simulink library "lib_energy_storage2"  (Simulink 4.1.1)
values from neighbouring files (symbols this model uses):
  logFlag = 1    [advSACompMaskInit.m]    (also in advSACompMaskInitR13.m)
undefined symbols (not defined in the file or in its folder): air_cp, amb_tmp, cyc_mph, enable_stop, ess_cap_scale, ess_cb, ess_cc, ess_coulombic_eff, ess_init_soc, ess_max_ah_cap, ess_max_p, ess_max_p_soc, ess_max_soc, ess_max_volts, ess_min_soc, ess_min_volts, ess_MMi, ess_MMo, ess_mod_airflow, ess_mod_cp, ess_mod_cpm, ess_mod_init_tmp, ess_module_mass, ess_module_num, ess_on, ess_parallel_mod_num, ess_res_scale_coef, ess_res_scale_fun, ess_set_tmp, ess_soc, ess_th_calc, ess_th_res, ess_th_res_off, ess_th_res_on, ess_tmp, ess_voc, fund_byu, fund_byuop, mc_min_volts, saber_air_temp, Saber_Battery_IO_File, saber_init_soc, saber_init_temp, saber_init_voc, saber_k_cb, saber_k_cc, saber_k_rc, saber_k_re, saber_k_rt, saber_k_soc, t_soc, time_step
libraries: simulink3 x16, lib_energy_storage x1, lib_energy_storage2 x1
(part 7 of 10)

== system lib_energy_storage2/energy storage <ess>/energy storage <ess>/Model/compute current ==
  Voc : Inport  Port=1  LatchInput=off
  Rint : Inport  Port=2  LatchInput=off
  limited output power (W) : Inport  Port=3  LatchInput=off
  Ibty=(Voc-(Voc^2-4RPbty)^.5)        ----------------------------- (2*R) : Fcn  Expr=(u[2]-(u[2]^2-4*u[1]*u[3])^.5)/(2*u[3])
  Logical Operator1 : Logic  Operator=NOT  Inputs=1
  Mux3 : Mux  Inputs=3
      settings: DisplayOption=none
  Mux4 : Mux  Inputs=3
      settings: DisplayOption=none
  Mux5 : Mux  Inputs=3
      settings: DisplayOption=none
  Voc-I*R : Fcn  Expr=u[2]-u[1]*u[3]
  enhancedToWorkspace2 : Subsystem  TreatAsAtomicUnit=on  mask(enhancedToWorkspace){generalName=generalName, specificName=current, logFlag=logFlag}
      mask prompts: generalName "General Name [char-evaluated]"; specificName "Specific Name [char-literal]"; logFlag "Enable flag (1=on,0=off)"
      mask help: A wrapper for the Simulink "To Workspace" block that allows you to evaluate the name of the variable to log to workspace. This is useful to avoid the double logging errors that occur when you pull in two library models that attempt to log to the same variable.
      mask init:
      | enhancedToWsMaker
      settings: CopyFcn=breakLinkCopyFcn  ParentCloseFcn=breakLinkParCloseFcn  RTWFcnNameOpts=Auto  RTWFileNameOpts=Auto
      mask Help:
      | <h2>Enhanced To Workspace Block</h2>
      | <h3>Parameters</h3>
      | <UL>
      | <li><b>General Name:</b> This is the more general name of the variable. Variables are saved to the workspace as <i>generalName_specificName</i>. Note that this is an evaluated variable. If you would like to type in the value directly, it must be surrounded with single quotes. Otherwise you can input the name of a variable containing a char string.</li>
      | <li><b>Specific Name:</b> This is the specific name of the variable. Note that this is input as a char literal (i.e., you don't need quotes).</li>
      | <li><b>Enable Flag:</b> This flag should have the value of 0 or 1. If 0, the variable will not be logged to the workspace. If 1, the variable will be logged. This is done so that variable logging can be turned off to improve speed.</li>
      | </ul>
      | <h3>Overview</h3>
      | <p>The enhanced to workspace block was put together to allow one to dynamically resolve variable names at run time in simulink. This is most powerful when used in conjunction with a masked subsystem to allow multiple instances of that masked subsytem to be used in the same model. The strategy is to set the generalName in the block mask which will allow the block to change the general name for all variable logging on the fly.
      | <h3>Helper Files</h3>
      | <p>Three m-files are required by the enhancedToWorkspace block. These files are located in the &lt; ADVISOR root &gt;/GUI directory :
      | <ul>
      | <li><i>enhancedToWsMaker.m</i> This file runs the mask initialization for the block</li>
      | <li><i>breakLinkCopyFcn.m</i> This file is used by the block callback when the simulink block is copied. It is necessary to break the link to the enhancedToWorkspace similar to the To Workspace block in order for it to be able to configure itself. (Try copying simulink's To Workspace block--it is impossible to make a link)</li>
      | <li><i>breakLinkParCloseFcn.m</i> This file is similar to the breakLinkCopyFcn and is used when a parent system is closed</li>
      | </ul>
      | <hr>
      | 
      | <p>Created 2003-Jan-21, Michael Patrick O'Keefe, NREL</p>
      | 
      | <!--
      | <VARDEF>
      | <H3>var_name</H3>
      | <UL>
      | <LI><B>data type</B> data type here</LI>
      | <LI><B>units</B> units here</LI>
      | <LI><B>vehicle type</B> vehicle type here</LI>
      | <LI><B>description</B> description here</LI>
      | </UL>
      | </VARDEF>
      | -->
      mask Display: disp([generalName,'_',specificName])
  ess max voltage*#batts : Constant  Value=ess_max_volts*ess_module_num
  iabs min=(Voc-Vmax)/R : Fcn  Expr=(u(1)-u(2))/u(3)
  limit current based on  max voltage during charge : Switch  Threshold=eps
  min charge current not exceeded : RelationalOperator  Operator=>
  I_ : Outport  Port=1  InitialOutput=0
  V_ : Outport  Port=2  InitialOutput=0
  tag scope: ess_maxV_limited=scoped
  wires:
  Logical Operator1/1 -> [ess_maxV_limited]
  ess max voltage*#batts/1 -> Mux5/2
  Mux5/1 -> iabs min=(Voc-Vmax)/R/1
  Mux4/1 -> Ibty=(Voc-(Voc^2-4RPbty)^.5)        ----------------------------- (2*R)/1
  Voc-I*R/1 -> V_/1
  Mux3/1 -> Voc-I*R/1
  min charge current not exceeded/1 -> Logical Operator1/1, limit current based on  max voltage during charge/2
  limit current based on  max voltage during charge/1 -> Mux3/1, I_/1, enhancedToWorkspace2/1(In1)
  iabs min=(Voc-Vmax)/R/1 -> limit current based on  max voltage during charge/3, min charge current not exceeded/2
  Ibty=(Voc-(Voc^2-4RPbty)^.5)        ----------------------------- (2*R)/1 -> limit current based on  max voltage during charge/1, min charge current not exceeded/1
  Rint/1 -> Mux5/3, Mux3/3, Mux4/3
  Voc/1 -> Mux5/1, Mux3/2, Mux4/2
  limited output power (W)/1 -> Mux4/1

== system lib_energy_storage2/energy storage <ess>/energy storage <ess>/Model/documentation9 ==

== system lib_energy_storage2/energy storage <ess>/energy storage <ess>/Model/enhancedToWorkspace ==
  In1 : Inport  Port=1  LatchInput=off
  Terminator : Terminator
  wires:
  In1/1 -> Terminator/1

== system lib_energy_storage2/energy storage <ess>/energy storage <ess>/Model/enhancedToWorkspace1 ==
  In1 : Inport  Port=1  LatchInput=off
  Terminator : Terminator
  wires:
  In1/1 -> Terminator/1

== system lib_energy_storage2/energy storage <ess>/energy storage <ess>/Model/enhancedToWorkspace2 ==
  In1 : Inport  Port=1  LatchInput=off
  Terminator : Terminator
  wires:
  In1/1 -> Terminator/1

== system lib_energy_storage2/energy storage <ess>/energy storage <ess>/Model/enhancedToWorkspace3 ==
  In1 : Inport  Port=1  LatchInput=off
  Terminator : Terminator
  wires:
  In1/1 -> Terminator/1

== system lib_energy_storage2/energy storage <ess>/energy storage <ess>/Model/enhancedToWorkspace4 ==
  In1 : Inport  Port=1  LatchInput=off
  Terminator : Terminator
  wires:
  In1/1 -> Terminator/1

== system lib_energy_storage2/energy storage <ess>/energy storage <ess>/Model/enhancedToWorkspace5 ==
  In1 : Inport  Port=1  LatchInput=off
  Terminator : Terminator
  wires:
  In1/1 -> Terminator/1

== system lib_energy_storage2/energy storage <ess>/energy storage <ess>/Model/ess tmp ==
  Qess_gen : Inport  Port=1  LatchInput=off
  Enable : EnablePort  StatesWhenEnabling=reset
  #of mods : Gain  Gain=ess_module_num  Multiplication=Element-wise(K.*u)  SaturateOnIntegerOverflow=on
  1/#of mods : Gain  Gain=1/ess_module_num  Multiplication=Element-wise(K.*u)  SaturateOnIntegerOverflow=on
  1/mcp : Gain  Gain=1/(ess_module_mass*ess_mod_cp)  Multiplication=Element-wise(K.*u)  SaturateOnIntegerOverflow=on
  Block NOTES : Subsystem
      settings: RTWFcnNameOpts=Auto  RTWFileNameOpts=Auto
      mask Display: disp('Block\nNOTES')
  Memory : Memory  Orientation=left  X0=cyc_mph(1,2)*.447  InheritSampleTime=off
      settings: RTWStateStorageClass=Auto
  Memory1 : Memory  Orientation=left  X0=cyc_mph(1,2)*.447  InheritSampleTime=off
      settings: RTWStateStorageClass=Auto
  Mux20 : Mux  Inputs=3
      settings: DisplayOption=none
  Qc : Sum  Inputs=++  SaturateOnIntegerOverflow=on
  Qess_case : Fcn  Expr=(u(2) - u(1))/u(3)
  Saturation3 : Saturate  Orientation=left  UpperLimit=1  LowerLimit=0  LinearizeAsGain=on
  Tair,ave : Subsystem  TreatAsAtomicUnit=on
      settings: RTWFcnNameOpts=Auto  RTWFileNameOpts=Auto
  Tess2 : Integrator  ExternalReset=none  InitialConditionSource=internal  InitialCondition=ess_mod_init_tmp  LimitOutput=off  UpperSaturationLimit=inf  LowerSaturationLimit=-inf  ShowSaturationPort=off  ShowStatePort=off  AbsoluteTolerance=auto
  thermostat : Fcn  Orientation=left  Expr=u(1) - ess_set_tmp
  Tess : Outport  Port=1  InitialOutput=0
  Tair : Outport  Port=2
  Qair : Outport  Port=3  OutputWhenDisabled=reset  InitialOutput=0
  wires:
  Tair,ave/1(Tair_ave) -> Tair/1, Mux20/2
  Tair,ave/2(Th Res) -> Mux20/3
  Mux20/1 -> Qess_case/1
  #of mods/1 -> Qair/1
  Memory/1 -> Tair,ave/1(Qess_case)
  Memory1/1 -> Tair,ave/Enable
  Saturation3/1 -> Memory1/1
  thermostat/1 -> Saturation3/1
  1/#of mods/1 -> Qc/2
  Qess_gen/1 -> 1/#of mods/1
  Tess2/1 -> thermostat/1, Mux20/1, Tess/1
  1/mcp/1 -> Tess2/1
  Qess_case/1 -> #of mods/1, Memory/1, Qc/1
  Qc/1 -> 1/mcp/1

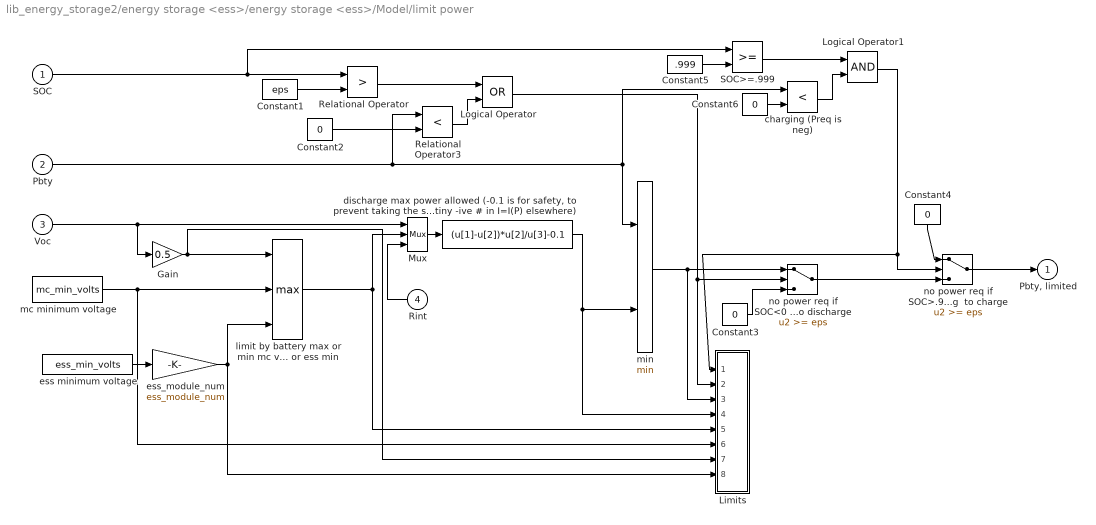
== system lib_energy_storage2/energy storage <ess>/energy storage <ess>/Model/limit power ==
  SOC : Inport  Port=1  LatchInput=off
  Pbty : Inport  Port=2  LatchInput=off
  Voc : Inport  Port=3  LatchInput=off
  Rint : Inport  Orientation=left  Port=4  LatchInput=off
  Constant1 : Constant  Value=eps
  Constant2 : Constant  Value=0
  Constant3 : Constant  Value=0
  Constant4 : Constant  Orientation=down  Value=0
  Constant5 : Constant  Value=.999
  Constant6 : Constant  Value=0
  Gain : Gain  Gain=0.5  Multiplication=Element-wise(K.*u)  SaturateOnIntegerOverflow=on
  Limits : Subsystem
      settings: RTWFcnNameOpts=Auto  RTWFileNameOpts=Auto
  Logical Operator : Logic  Operator=OR  Inputs=2
  Logical Operator1 : Logic  Operator=AND  Inputs=2
  Mux : Mux  Inputs=3
      settings: DisplayOption=none
  Relational Operator : RelationalOperator  Operator=>
  Relational Operator3 : RelationalOperator  Operator=<
  SOC>=.999 : RelationalOperator  Operator=>=
  charging (Preq is neg) : RelationalOperator  Operator=<
  "discharge max power allowed (-0.1 is for safety, to prevent taking the square of a tiny -ive # in I=I(P) elsewhere)" : Fcn  Expr=(u[1]-u[2])*u[2]/u[3]-0.1
  ess minimum voltage : Constant  Value=ess_min_volts
  ess_module_num : Gain  Gain=ess_module_num  Multiplication=Element-wise(K.*u)  SaturateOnIntegerOverflow=on
  limit by battery max or min mc voltage or ess min : MinMax  Function=max  Inputs=3
  mc minimum voltage : Constant  Value=mc_min_volts
  min : MinMax  Function=min  Inputs=2
  no power req if SOC<0 and trying  to discharge : Switch  Threshold=eps
  no power req if SOC>.999 and trying  to charge : Switch  Threshold=eps
  "Pbty, limited" : Outport  Port=1  InitialOutput=0
  wires:
  Logical Operator1/1 -> Limits/1(SOC  high limited), no power req if SOC>.999 and trying  to charge/2
  no power req if SOC>.999 and trying  to charge/1 -> "Pbty, limited"/1
  no power req if SOC<0 and trying  to discharge/1 -> no power req if SOC>.999 and trying  to charge/3
  Constant4/1 -> no power req if SOC>.999 and trying  to charge/1
  Constant5/1 -> SOC>=.999/2
  charging (Preq is neg)/1 -> Logical Operator1/2
  Constant6/1 -> charging (Preq is neg)/2
  SOC>=.999/1 -> Logical Operator1/1
  SOC/1 -> SOC>=.999/1, Relational Operator/1
  ess_module_num/1 -> Limits/8(V ess_min_volts), limit by battery max or min mc voltage or ess min/3
  ess minimum voltage/1 -> ess_module_num/1
  Gain/1 -> Limits/7(V battery (.5Voc)), limit by battery max or min mc voltage or ess min/1
  Rint/1 -> Mux/3
  mc minimum voltage/1 -> Limits/6(V mc_min_volts), limit by battery max or min mc voltage or ess min/2
  "discharge max power allowed (-0.1 is for safety, to prevent taking the square of a tiny -ive # in I=I(P) elsewhere)"/1 -> min/2, Limits/4(power bat limited)
  limit by battery max or min mc voltage or ess min/1 -> Limits/5(V used), Mux/2
  Mux/1 -> "discharge max power allowed (-0.1 is for safety, to prevent taking the square of a tiny -ive # in I=I(P) elsewhere)"/1
  min/1 -> Limits/3(power req), no power req if SOC<0 and trying  to discharge/1
  Voc/1 -> Gain/1, Mux/1
  Logical Operator/1 -> Limits/2(not SOC  low limited), no power req if SOC<0 and trying  to discharge/2
  Constant3/1 -> no power req if SOC<0 and trying  to discharge/3
  Relational Operator3/1 -> Logical Operator/2
  Constant2/1 -> Relational Operator3/2
  Pbty/1 -> charging (Preq is neg)/1, min/1, Relational Operator3/1
  Relational Operator/1 -> Logical Operator/1
  Constant1/1 -> Relational Operator/2

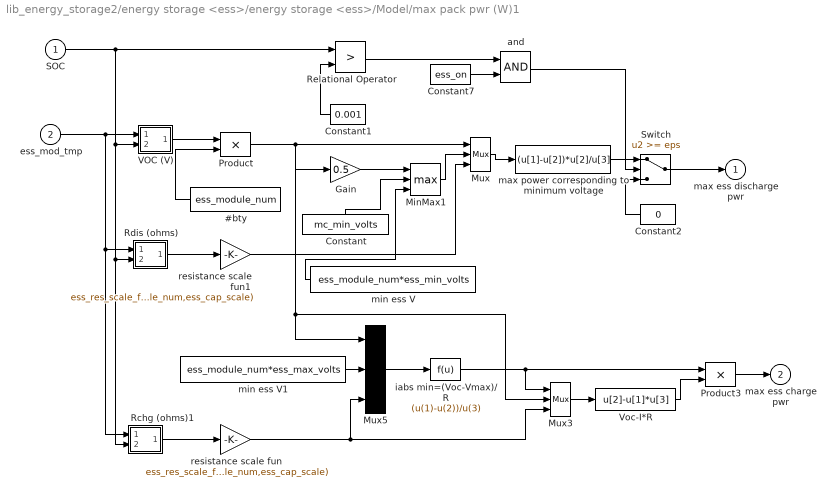
== system lib_energy_storage2/energy storage <ess>/energy storage <ess>/Model/max pack pwr (W)1 ==
  SOC : Inport  Port=1  LatchInput=off
  ess_mod_tmp : Inport  Port=2  LatchInput=off
  #bty : Constant  Orientation=left  Value=ess_module_num
  Constant : Constant  Orientation=up  Value=mc_min_volts
  Constant1 : Constant  Orientation=left  Value=0.001
  Constant2 : Constant  Orientation=left  Value=0
  Constant7 : Constant  Value=ess_on
  Gain : Gain  Gain=0.5  Multiplication=Element-wise(K.*u)  SaturateOnIntegerOverflow=on
  MinMax1 : MinMax  Function=max  Inputs=3
  Mux : Mux  Inputs=3
      settings: DisplayOption=none
  Mux3 : Mux  Inputs=3
      settings: DisplayOption=none
  Mux5 : Mux  Inputs=3
      settings: DisplayOption=none
  Product : Product  Inputs=2  Multiplication=Element-wise(.*)  SaturateOnIntegerOverflow=on
  Product3 : Product  Inputs=2  Multiplication=Element-wise(.*)  SaturateOnIntegerOverflow=on
  Rchg (ohms)1 : Subsystem  mask(2-D Table Lookup){@1=ess_tmp, @2=ess_soc, @3=ess_r_chg}
      mask prompts: @1 "X Index"; @2 "Y Index"; @3 "Table"
      mask help:
      | Two Dimensional Table Lookup
      | The first input corresponds to X Index and the second input corresponds to the Y Index
      mask init:
      | xindex=@1; yindex=@2; table=@3; sftab2chk(xindex,yindex,table);
      settings: RTWFcnNameOpts=Auto  RTWFileNameOpts=Auto
      mask Help: This block returns a linearly interpolated intersection from the table using the X index (which corresponds to the rows of the table) and the Y index (which corresponds to the columns of the table).  Extrapolation is used.
      mask Display: plot(-10,-10,110,110,[90,50,10],[90,40,30],[90,50,10],[50,26,20],[90,50,10],[22,13,10])
  Rdis (ohms) : Subsystem  mask(2-D Table Lookup){@1=ess_tmp, @2=ess_soc, @3=ess_r_dis}
      mask prompts: @1 "X Index"; @2 "Y Index"; @3 "Table"
      mask help:
      | Two Dimensional Table Lookup
      | The first input corresponds to X Index and the second input corresponds to the Y Index
      mask init:
      | xindex=@1; yindex=@2; table=@3; sftab2chk(xindex,yindex,table);
      settings: RTWFcnNameOpts=Auto  RTWFileNameOpts=Auto
      mask Help: This block returns a linearly interpolated intersection from the table using the X index (which corresponds to the rows of the table) and the Y index (which corresponds to the columns of the table).  Extrapolation is used.
      mask Display: plot(-10,-10,110,110,[90,50,10],[90,40,30],[90,50,10],[50,26,20],[90,50,10],[22,13,10])
  Relational Operator : RelationalOperator  Operator=>
  Switch : Switch  Threshold=eps
  VOC (V) : Subsystem  mask(2-D Table Lookup){@1=ess_tmp, @2=ess_soc, @3=ess_voc}
      mask prompts: @1 "X Index"; @2 "Y Index"; @3 "Table"
      mask help:
      | Two Dimensional Table Lookup
      | The first input corresponds to X Index and the second input corresponds to the Y Index
      mask init:
      | xindex=@1; yindex=@2; table=@3; sftab2chk(xindex,yindex,table);
      settings: RTWFcnNameOpts=Auto  RTWFileNameOpts=Auto
      mask Help: This block returns a linearly interpolated intersection from the table using the X index (which corresponds to the rows of the table) and the Y index (which corresponds to the columns of the table).  Extrapolation is used.
      mask Display: plot(-10,-10,110,110,[90,50,10],[90,40,30],[90,50,10],[50,26,20],[90,50,10],[22,13,10])
  Voc-I*R : Fcn  Expr=u[2]-u[1]*u[3]
  and : Logic  Operator=AND  Inputs=2
  iabs min=(Voc-Vmax)/R : Fcn  Expr=(u(1)-u(2))/u(3)
  max power corresponding to minimum voltage : Fcn  Expr=(u[1]-u[2])*u[2]/u[3]
  min ess V : Constant  Orientation=left  Value=ess_module_num*ess_min_volts
  min ess V1 : Constant  Value=ess_module_num*ess_max_volts
  resistance scale fun : Gain  Gain=ess_res_scale_fun(ess_res_scale_coef,ess_module_num,ess_cap_scale)  Multiplication=Element-wise(K.*u)  SaturateOnIntegerOverflow=on
  resistance scale fun1 : Gain  Gain=ess_res_scale_fun(ess_res_scale_coef,ess_module_num,ess_cap_scale)  Multiplication=Element-wise(K.*u)  SaturateOnIntegerOverflow=on
  max ess discharge pwr : Outport  Port=1  InitialOutput=0
  max ess charge pwr : Outport  Port=2  InitialOutput=0
  wires:
  Constant7/1 -> and/2
  Relational Operator/1 -> and/1
  and/1 -> Switch/2
  min ess V/1 -> MinMax1/3
  ess_mod_tmp/1 -> VOC (V)/1(x0), Rdis (ohms)/1(x0), Rchg (ohms)1/1(x0)
  Constant1/1 -> Relational Operator/2
  Constant/1 -> MinMax1/2
  Mux/1 -> max power corresponding to minimum voltage/1
  Gain/1 -> MinMax1/1
  MinMax1/1 -> Mux/2
  Product/1 -> Mux/1, Gain/1, Mux5/1, Mux3/2
  resistance scale fun1/1 -> Mux/3
  VOC (V)/1(table out) -> Product/1
  Rdis (ohms)/1(table out) -> resistance scale fun1/1
  max power corresponding to minimum voltage/1 -> Switch/1
  Constant2/1 -> Switch/3
  SOC/1 -> Relational Operator/1, VOC (V)/2(y0), Rdis (ohms)/2(y0), Rchg (ohms)1/2(y0)
  Switch/1 -> max ess discharge pwr/1
  min ess V1/1 -> Mux5/2
  Mux5/1 -> iabs min=(Voc-Vmax)/R/1
  Mux3/1 -> Voc-I*R/1
  iabs min=(Voc-Vmax)/R/1 -> Mux3/1, Product3/1
  Voc-I*R/1 -> Product3/2
  Product3/1 -> max ess charge pwr/1
  resistance scale fun/1 -> Mux5/3, Mux3/3
  Rchg (ohms)1/1(table out) -> resistance scale fun/1
  #bty/1 -> Product/2

== system lib_energy_storage2/energy storage <ess>/energy storage <ess>/Model/pack Voc, Rint ==
  SOC (prev) : Inport  Port=1  LatchInput=off
  req'd battery power (W) : Inport  Port=2  LatchInput=off
  mod tmp   (C) : Inport  Port=3  LatchInput=off
  #bty : Constant  Value=ess_module_num
  Product : Product  Inputs=2  Multiplication=Element-wise(.*)  SaturateOnIntegerOverflow=on
  Rchg (ohms) : Subsystem  mask(2-D Table Lookup){@1=ess_tmp, @2=ess_soc, @3=ess_r_chg}
      mask prompts: @1 "X Index"; @2 "Y Index"; @3 "Table"
      mask help:
      | Two Dimensional Table Lookup
      | The first input corresponds to X Index and the second input corresponds to the Y Index
      mask init:
      | xindex=@1; yindex=@2; table=@3; sftab2chk(xindex,yindex,table);
      settings: RTWFcnNameOpts=Auto  RTWFileNameOpts=Auto
      mask Help: This block returns a linearly interpolated intersection from the table using the X index (which corresponds to the rows of the table) and the Y index (which corresponds to the columns of the table).  Extrapolation is used.
      mask Display: plot(-10,-10,110,110,[90,50,10],[90,40,30],[90,50,10],[50,26,20],[90,50,10],[22,13,10])
  Rdis (ohms) : Subsystem  mask(2-D Table Lookup){@1=ess_tmp, @2=ess_soc, @3=ess_r_dis}
      mask prompts: @1 "X Index"; @2 "Y Index"; @3 "Table"
      mask help:
      | Two Dimensional Table Lookup
      | The first input corresponds to X Index and the second input corresponds to the Y Index
      mask init:
      | xindex=@1; yindex=@2; table=@3; sftab2chk(xindex,yindex,table);
      settings: RTWFcnNameOpts=Auto  RTWFileNameOpts=Auto
      mask Help: This block returns a linearly interpolated intersection from the table using the X index (which corresponds to the rows of the table) and the Y index (which corresponds to the columns of the table).  Extrapolation is used.
      mask Display: plot(-10,-10,110,110,[90,50,10],[90,40,30],[90,50,10],[50,26,20],[90,50,10],[22,13,10])
  Switch : Switch  Threshold=0
  VOC (V) : Subsystem  mask(2-D Table Lookup){@1=ess_tmp, @2=ess_soc, @3=ess_voc}
      mask prompts: @1 "X Index"; @2 "Y Index"; @3 "Table"
      mask help:
      | Two Dimensional Table Lookup
      | The first input corresponds to X Index and the second input corresponds to the Y Index
      mask init:
      | xindex=@1; yindex=@2; table=@3; sftab2chk(xindex,yindex,table);
      settings: RTWFcnNameOpts=Auto  RTWFileNameOpts=Auto
      mask Help: This block returns a linearly interpolated intersection from the table using the X index (which corresponds to the rows of the table) and the Y index (which corresponds to the columns of the table).  Extrapolation is used.
      mask Display: plot(-10,-10,110,110,[90,50,10],[90,40,30],[90,50,10],[50,26,20],[90,50,10],[22,13,10])
  resistance scale fun : Gain  Gain=ess_res_scale_fun(ess_res_scale_coef,ess_module_num,ess_cap_scale)  Multiplication=Element-wise(K.*u)  SaturateOnIntegerOverflow=on
  resistance scale fun1 : Gain  Gain=ess_res_scale_fun(ess_res_scale_coef,ess_module_num,ess_cap_scale)  Multiplication=Element-wise(K.*u)  SaturateOnIntegerOverflow=on
  pack open- circuit voltage : Outport  Port=1  InitialOutput=0
  pack resistance : Outport  Port=2  InitialOutput=0
  wires:
  mod tmp   (C)/1 -> Rchg (ohms)/1(x0), Rdis (ohms)/1(x0), VOC (V)/1(x0)
  SOC (prev)/1 -> Rchg (ohms)/2(y0), Rdis (ohms)/2(y0), VOC (V)/2(y0)
  req'd battery power (W)/1 -> Switch/2
  VOC (V)/1(table out) -> Product/1
  Product/1 -> pack open- circuit voltage/1
  #bty/1 -> Product/2
  Switch/1 -> pack resistance/1
  Rdis (ohms)/1(table out) -> resistance scale fun/1
  resistance scale fun/1 -> Switch/1
  Rchg (ohms)/1(table out) -> resistance scale fun1/1
  resistance scale fun1/1 -> Switch/3

== system lib_energy_storage2/energy storage <ess>/energy storage <ess>/Model/stop sim ==
  SOC : Inport  Port=1  LatchInput=off
  Enable : EnablePort
  Const : Constant  Orientation=up  Value=.001
  Relational Operator : RelationalOperator  Operator=<
  Stop Simulation : Stop
  wires:
  Relational Operator/1 -> Stop Simulation/1
  SOC/1 -> Relational Operator/1
  Const/1 -> Relational Operator/2

== system lib_energy_storage2/energy storage <ess> RC/energy storage <ess> RC/model/Allow simulation to stop based on  low SOC ==
  SOC : Inport  Port=1  LatchInput=off
  Enable : EnablePort
  Const : Constant  Orientation=up  Value=.001
  Relational Operator : RelationalOperator  Operator=<
  Stop Simulation : Stop
  wires:
  Relational Operator/1 -> Stop Simulation/1
  SOC/1 -> Relational Operator/1
  Const/1 -> Relational Operator/2

== system lib_energy_storage2/energy storage <ess> RC/energy storage <ess> RC/model/Block NOTES ==
  note: This block models the energy storage system as an SOC-dependent voltage
      | in series with an SOC- and current direction-dependent internal resistance.
      | SOC is computed assuming that A-h capacity is constant, but limited
      | such that a minimum voltage is never exceeded (replacing the
      | previous Peukert relationship which underpredicted battery capacity).
      |
      | Discharge power is limited here so as not to bring the bus (battery pack) voltage below
      | the minimum controller voltage or the minimum battery voltage and so as to allow
      | the solution of the quadratic eq'n for discharge current.
      |
      | Charge current is limited to ensure the voltage does not exceed a maximum
      | voltage
      |
      | Positive current is discharge current in the convention used here.
      | Power loss is computed as I*R+losses due to Coulombic (in)efficiency.
      |
      | Thermal modeling of the battery performance is modeled in the
      | OCV, Rint, and capacity.

== system lib_energy_storage2/energy storage <ess> RC/energy storage <ess> RC/model/Model Parameters ==
  SOC : Inport  Port=1  LatchInput=off
  Ess Temp : Inport  Port=2  LatchInput=off
  Preq : Inport  Port=3  LatchInput=off
  Terminator : Terminator
  cb : Lookup  InputValues=ess_tmp  OutputValues=ess_cb
  cc : Lookup  InputValues=ess_tmp  OutputValues=ess_cc
  rc : Subsystem  mask(2-D Table Lookup){@1=ess_tmp, @2=ess_soc, @3=ess_rc}
      mask prompts: @1 "X Index"; @2 "Y Index"; @3 "Table"
      mask help:
      | Two Dimensional Table Lookup
      | The first input corresponds to X Index and the second input corresponds to the Y Index
      mask init:
      | xindex=@1; yindex=@2; table=@3; sftab2chk(xindex,yindex,table);
      settings: RTWFcnNameOpts=Auto  RTWFileNameOpts=Auto
      mask Help: This block returns a linearly interpolated intersection from the table using the X index (which corresponds to the rows of the table) and the Y index (which corresponds to the columns of the table).  Extrapolation is used.
      mask Display: plot(-10,-10,110,110,[90,50,10],[90,40,30],[90,50,10],[50,26,20],[90,50,10],[22,13,10])
  re : Subsystem  mask(2-D Table Lookup){@1=ess_tmp, @2=ess_soc, @3=ess_re}
      mask prompts: @1 "X Index"; @2 "Y Index"; @3 "Table"
      mask help:
      | Two Dimensional Table Lookup
      | The first input corresponds to X Index and the second input corresponds to the Y Index
      mask init:
      | xindex=@1; yindex=@2; table=@3; sftab2chk(xindex,yindex,table);
      settings: RTWFcnNameOpts=Auto  RTWFileNameOpts=Auto
      mask Help: This block returns a linearly interpolated intersection from the table using the X index (which corresponds to the rows of the table) and the Y index (which corresponds to the columns of the table).  Extrapolation is used.
      mask Display: plot(-10,-10,110,110,[90,50,10],[90,40,30],[90,50,10],[50,26,20],[90,50,10],[22,13,10])
  rt : Subsystem  mask(2-D Table Lookup){@1=ess_tmp, @2=ess_soc, @3=ess_rt}
      mask prompts: @1 "X Index"; @2 "Y Index"; @3 "Table"
      mask help:
      | Two Dimensional Table Lookup
      | The first input corresponds to X Index and the second input corresponds to the Y Index
      mask init:
      | xindex=@1; yindex=@2; table=@3; sftab2chk(xindex,yindex,table);
      settings: RTWFcnNameOpts=Auto  RTWFileNameOpts=Auto
      mask Help: This block returns a linearly interpolated intersection from the table using the X index (which corresponds to the rows of the table) and the Y index (which corresponds to the columns of the table).  Extrapolation is used.
      mask Display: plot(-10,-10,110,110,[90,50,10],[90,40,30],[90,50,10],[50,26,20],[90,50,10],[22,13,10])
  Cb : Outport  Port=1  InitialOutput=0
  Cc : Outport  Port=2  InitialOutput=0
  Re : Outport  Port=3  InitialOutput=0
  Rc : Outport  Port=4  InitialOutput=0
  Rt : Outport  Port=5  InitialOutput=0
  wires:
  rc/1(table out) -> Rc/1
  rt/1(table out) -> Rt/1
  re/1(table out) -> Re/1
  cc/1 -> Cc/1
  cb/1 -> Cb/1
  SOC/1 -> rt/2(y0), rc/2(y0), re/2(y0)
  Preq/1 -> Terminator/1
  Ess Temp/1 -> rt/1(x0), rc/1(x0), re/1(x0), cc/1, cb/1

== system lib_energy_storage2/energy storage <ess> RC/energy storage <ess> RC/model/RC model ==
  Cb : Inport  Port=1  LatchInput=off
  Cc : Inport  Port=2  LatchInput=off
  Re : Inport  Port=3  LatchInput=off
  Rc : Inport  Port=4  LatchInput=off
  Rt : Inport  Port=5  LatchInput=off
  Preq : Inport  Port=6  LatchInput=off
  Ess Temp : Inport  Port=7  LatchInput=off
  #mods{,1..4} (5 alike) : Gain  Gain=ess_module_num  Multiplication=Element-wise(K.*u)  SaturateOnIntegerOverflow=on
  1/#mods : Gain  Gain=1/ess_module_num  Multiplication=Element-wise(K.*u)  SaturateOnIntegerOverflow=on
  Demux1 : Demux  Outputs=7  BusSelectionMode=off
  Memory1 : Memory  X0=ess_init_soc  InheritSampleTime=off
      settings: RTWStateStorageClass=Auto
  Memory2 : Memory  X0=0  InheritSampleTime=off
      settings: RTWStateStorageClass=Auto
  Memory3 : Memory  X0=0  InheritSampleTime=off
      settings: RTWStateStorageClass=Auto
  Mux2 : Mux  Inputs=7
      settings: DisplayOption=none
  RC model of one module : S-Function  FunctionName=RC  Parameters=ess_min_volts,ess_max_volts,mc_min_volts/ess_module_num,ess_soc,ess_tmp,ess_voc,ess_init_soc,ess_mod_init_tmp  PortCounts=[]  SFunctionModules=''
  enhancedToWorkspace6 : Subsystem  TreatAsAtomicUnit=on  mask(enhancedToWorkspace){generalName=generalName, specificName=current, logFlag=logFlag}
      mask prompts: generalName "General Name [char-evaluated]"; specificName "Specific Name [char-literal]"; logFlag "Enable flag (1=on,0=off)"
      mask help: A wrapper for the Simulink "To Workspace" block that allows you to evaluate the name of the variable to log to workspace. This is useful to avoid the double logging errors that occur when you pull in two library models that attempt to log to the same variable.
      mask init:
      | enhancedToWsMaker
      settings: CopyFcn=breakLinkCopyFcn  ParentCloseFcn=breakLinkParCloseFcn  RTWFcnNameOpts=Auto  RTWFileNameOpts=Auto
      mask Help:
      | <h2>Enhanced To Workspace Block</h2>
      | <h3>Parameters</h3>
      | <UL>
      | <li><b>General Name:</b> This is the more general name of the variable. Variables are saved to the workspace as <i>generalName_specificName</i>. Note that this is an evaluated variable. If you would like to type in the value directly, it must be surrounded with single quotes. Otherwise you can input the name of a variable containing a char string.</li>
      | <li><b>Specific Name:</b> This is the specific name of the variable. Note that this is input as a char literal (i.e., you don't need quotes).</li>
      | <li><b>Enable Flag:</b> This flag should have the value of 0 or 1. If 0, the variable will not be logged to the workspace. If 1, the variable will be logged. This is done so that variable logging can be turned off to improve speed.</li>
      | </ul>
      | <h3>Overview</h3>
      | <p>The enhanced to workspace block was put together to allow one to dynamically resolve variable names at run time in simulink. This is most powerful when used in conjunction with a masked subsystem to allow multiple instances of that masked subsytem to be used in the same model. The strategy is to set the generalName in the block mask which will allow the block to change the general name for all variable logging on the fly.
      | <h3>Helper Files</h3>
      | <p>Three m-files are required by the enhancedToWorkspace block. These files are located in the &lt; ADVISOR root &gt;/GUI directory :
      | <ul>
      | <li><i>enhancedToWsMaker.m</i> This file runs the mask initialization for the block</li>
      | <li><i>breakLinkCopyFcn.m</i> This file is used by the block callback when the simulink block is copied. It is necessary to break the link to the enhancedToWorkspace similar to the To Workspace block in order for it to be able to configure itself. (Try copying simulink's To Workspace block--it is impossible to make a link)</li>
      | <li><i>breakLinkParCloseFcn.m</i> This file is similar to the breakLinkCopyFcn and is used when a parent system is closed</li>
      | </ul>
      | <hr>
      | 
      | <p>Created 2003-Jan-21, Michael Patrick O'Keefe, NREL</p>
      | 
      | <!--
      | <VARDEF>
      | <H3>var_name</H3>
      | <UL>
      | <LI><B>data type</B> data type here</LI>
      | <LI><B>units</B> units here</LI>
      | <LI><B>vehicle type</B> vehicle type here</LI>
      | <LI><B>description</B> description here</LI>
      | </UL>
      | </VARDEF>
      | -->
      mask Display: disp([generalName,'_',specificName])
  Pavailable : Outport  Port=1  InitialOutput=0
  SOC : Outport  Port=2  InitialOutput=0
  Vout : Outport  Port=3  InitialOutput=0
  Qess_gen : Outport  Port=4  InitialOutput=0
  tag scope: ess_max_chg_pwr=scoped, ess_max_pwr=scoped
  wires:
  RC model of one module/1 -> Demux1/1
  #mods2/1 -> Qess_gen/1
  Demux1/4 -> #mods2/1
  #mods1/1 -> Vout/1
  Demux1/3 -> #mods1/1
  #mods/1 -> Pavailable/1
  Demux1/1 -> #mods/1
  1/#mods/1 -> Mux2/6
  Preq/1 -> 1/#mods/1
  Mux2/1 -> RC model of one module/1
  Rt/1 -> Mux2/5
  Rc/1 -> Mux2/4
  Re/1 -> Mux2/3
  Cc/1 -> Mux2/2
  Cb/1 -> Mux2/1
  Ess Temp/1 -> Mux2/7
  Demux1/7 -> enhancedToWorkspace6/1(In1)
  Demux1/6 -> #mods4/1
  Memory2/1 -> [ess_max_chg_pwr]
  Demux1/5 -> #mods3/1
  Memory3/1 -> [ess_max_pwr]
  Demux1/2 -> Memory1/1
  Memory1/1 -> SOC/1
  #mods3/1 -> Memory3/1
  #mods4/1 -> Memory2/1

== system lib_energy_storage2/energy storage <ess> RC/energy storage <ess> RC/model/Thermal Model of Battery ==
  Qess_gen : Inport  Port=1  LatchInput=off
  Enable : EnablePort  StatesWhenEnabling=reset
  #of mods : Gain  Gain=ess_module_num  Multiplication=Element-wise(K.*u)  SaturateOnIntegerOverflow=on
  1/#of mods : Gain  Gain=1/ess_module_num  Multiplication=Element-wise(K.*u)  SaturateOnIntegerOverflow=on
  1/mcp : Gain  Gain=1/(ess_module_mass*ess_mod_cp)  Multiplication=Element-wise(K.*u)  SaturateOnIntegerOverflow=on
  Block NOTES : Subsystem
      settings: RTWFcnNameOpts=Auto  RTWFileNameOpts=Auto
      mask Display: disp('Block\nNOTES')
  Memory : Memory  Orientation=left  X0=cyc_mph(1,2)*.447  InheritSampleTime=off
      settings: RTWStateStorageClass=Auto
  Memory1 : Memory  Orientation=left  X0=cyc_mph(1,2)*.447  InheritSampleTime=off
      settings: RTWStateStorageClass=Auto
  Mux20 : Mux  Inputs=3
      settings: DisplayOption=none
  Qc : Sum  Inputs=++  SaturateOnIntegerOverflow=on
  Qess_case : Fcn  Expr=(u(2) - u(1))/u(3)
  Saturation3 : Saturate  Orientation=left  UpperLimit=1  LowerLimit=0  LinearizeAsGain=on
  Tair,ave : Subsystem  TreatAsAtomicUnit=on
      settings: RTWFcnNameOpts=Auto  RTWFileNameOpts=Auto
  Tess2 : Integrator  ExternalReset=none  InitialConditionSource=internal  InitialCondition=ess_mod_init_tmp  LimitOutput=off  UpperSaturationLimit=inf  LowerSaturationLimit=-inf  ShowSaturationPort=off  ShowStatePort=off  AbsoluteTolerance=auto
  thermostat : Fcn  Orientation=left  Expr=u(1) - ess_set_tmp
  Tess : Outport  Port=1  InitialOutput=0
  Tair : Outport  Port=2
  Qair : Outport  Port=3  OutputWhenDisabled=reset  InitialOutput=0
  wires:
  Tair,ave/1(Tair_ave) -> Tair/1, Mux20/2
  Tair,ave/2(Th Res) -> Mux20/3
  Mux20/1 -> Qess_case/1
  #of mods/1 -> Qair/1
  Memory/1 -> Tair,ave/1(Qess_case)
  Memory1/1 -> Tair,ave/Enable
  Saturation3/1 -> Memory1/1
  thermostat/1 -> Saturation3/1
  1/#of mods/1 -> Qc/2
  Qess_gen/1 -> 1/#of mods/1
  Tess2/1 -> thermostat/1, Mux20/1, Tess/1
  1/mcp/1 -> Tess2/1
  Qess_case/1 -> #of mods/1, Memory/1, Qc/1
  Qc/1 -> 1/mcp/1

== system lib_energy_storage2/energy storage <ess> RC/energy storage <ess> RC/model/documentation9 ==

== system lib_energy_storage2/energy storage <ess> RC/energy storage <ess> RC/model/enhancedToWorkspace ==
  In1 : Inport  Port=1  LatchInput=off
  Terminator : Terminator
  wires:
  In1/1 -> Terminator/1

== system lib_energy_storage2/energy storage <ess> RC/energy storage <ess> RC/model/enhancedToWorkspace1 ==
  In1 : Inport  Port=1  LatchInput=off
  Terminator : Terminator
  wires:
  In1/1 -> Terminator/1

== system lib_energy_storage2/energy storage <ess> RC/energy storage <ess> RC/model/enhancedToWorkspace2 ==
  In1 : Inport  Port=1  LatchInput=off
  Terminator : Terminator
  wires:
  In1/1 -> Terminator/1

== system lib_energy_storage2/energy storage <ess> RC/energy storage <ess> RC/model/enhancedToWorkspace3 ==
  In1 : Inport  Port=1  LatchInput=off
  Terminator : Terminator
  wires:
  In1/1 -> Terminator/1

== system lib_energy_storage2/energy storage <ess> RC/energy storage <ess> RC/model/enhancedToWorkspace4 ==
  In1 : Inport  Port=1  LatchInput=off
  Terminator : Terminator
  wires:
  In1/1 -> Terminator/1

== system lib_energy_storage2/energy storage <ess> RC/energy storage <ess> RC/model/enhancedToWorkspace5 ==
  In1 : Inport  Port=1  LatchInput=off
  Terminator : Terminator
  wires:
  In1/1 -> Terminator/1

== system lib_energy_storage2/energy storage <ess> RC/energy storage <ess> RC/model/enhancedToWorkspace6 ==
  In1 : Inport  Port=1  LatchInput=off
  Terminator : Terminator
  wires:
  In1/1 -> Terminator/1

== system lib_energy_storage2/energy storage <ess> nnet/energy storage <ess> nnet/model/Limits ==
  power req : Inport  Port=1  LatchInput=off
  power  available from battery : Inport  Port=2  LatchInput=off
  Const{1..4} (4 alike) : Constant  Value=0
  Relational Operator1 : RelationalOperator  Operator===
  limited by battery : Logic  Operator=NOT  Inputs=1
  tag scope: ess_maxV_limited=scoped, ess_minV_limited=scoped, ess_pwr_limited=scoped, ess_soc_limited=scoped, mc_voltage_limited=scoped
  wires:
  Relational Operator1/1 -> limited by battery/1
  limited by battery/1 -> [ess_pwr_limited]
  power req/1 -> Relational Operator1/1
  power  available from battery/1 -> Relational Operator1/2
  Const4/1 -> [mc_voltage_limited]
  Const3/1 -> [ess_minV_limited]
  Const2/1 -> [ess_maxV_limited]
  Const1/1 -> [ess_soc_limited]

== system lib_energy_storage2/energy storage <ess> nnet/energy storage <ess> nnet/model/NNet ==
  Preq : Inport  Port=1  LatchInput=off
  SOC : Inport  Port=2  LatchInput=off
  Enable : EnablePort
  De-Normalizer1 Voltage : Fcn  Expr=(u-0.2)*(ess_MMo(2,2)-ess_MMo(2,1))/(0.8-0.2)+ess_MMo(2,1)
  De-Normalizer2 Current : Fcn  Expr=(u-0.2)*(ess_MMo(1,2)-ess_MMo(1,1))/(0.8-0.2)+ess_MMo(1,1)
  Demux : Demux  Outputs=2  BusSelectionMode=off
  Mux : Mux  Inputs=2
      settings: DisplayOption=none
  Neural Network : Subsystem
      settings: RTWFcnNameOpts=Auto  RTWFileNameOpts=Auto
  Normalizer Power : Fcn  Expr=(u-ess_MMi(1,1))/(ess_MMi(1,2)-ess_MMi(1,1))
  Normalizer SOC : Fcn  Expr=(u-ess_MMi(2,1))/(ess_MMi(2,2)-ess_MMi(2,1))
  V : Outport  Port=1  InitialOutput=0
  i : Outport  Port=2  OutputWhenDisabled=reset  InitialOutput=0
  wires:
  De-Normalizer1 Voltage/1 -> V/1
  Demux/2 -> De-Normalizer1 Voltage/1
  Demux/1 -> De-Normalizer2 Current/1
  De-Normalizer2 Current/1 -> i/1
  Normalizer SOC/1 -> Mux/2
  SOC/1 -> Normalizer SOC/1
  Normalizer Power/1 -> Mux/1
  Preq/1 -> Normalizer Power/1
  Neural Network/1("y{1}") -> Demux/1
  Mux/1 -> Neural Network/1("p{1}")
